simulink model "mdaqdemos_rc_controller"  (R2013a)
settings: Solver=FixedStepDiscrete  SolverMode=SingleTasking  StartTime=0.0  StopTime=inf  FixedStep=0.001  RelTol=1e-3
libraries: microdaq_lib x2
settings Model: SimulationMode=external  Creator=skibool  LastModifiedBy=skibool
settings OptimizationCC: OptimizeModelRefInitCode=on  LifeSpan=1
settings DebuggingCC: UnderspecifiedInitializationDetection=Simplified  StateNameClashWarn=none
settings HardwareCC: ProdBitPerLong=40  ProdLargestAtomicInteger=Integer  ProdIntDivRoundTo=Zero  ProdEndianess=LittleEndian  ProdHWDeviceType=Texas Instruments->C6000
settings RTWCC: SystemTargetFile=microdaq.tlc  TemplateMakefile=microdaq.tmf  PostCodeGenCommand=microdaq_postcodegen(buildInfo)  Description=MicroDAQ Real-Time Measurement System  ProcessScript=microdaq_make_rtw_hook
settings CodeAppCC: IgnoreCustomStorageClasses=off
settings STFCustomTargetCC: CodeReplacementLibrary=TI C674x  CombineOutputUpdateFcns=on  ERTCustomFileBanners=on  SupportContinuousTime=off  SupportNonInlinedSFcns=off  MATLABClassNameForMDSCustomization=Simulink.SoftwareTarget.ERTCustomization  SystemTargetFile=microdaq.tlc
settings ERTTargetCC: CodeReplacementLibrary=TI C674x  GenerateSampleERTMain=off  ParMdlRefBuildCompliant=off  CompOptLevelCompliant=off  ConcurrentExecutionCompliant=off  ERTFirstTimeCompliant=off  ModelStepFunctionPrototypeControlCompliant=off  CPPClassGenCompliant=off  ExtMode=on  ExtModeStaticAlloc=on  ExtModeStaticAllocSize=10485760  ExtModeMexArgs=getpref('microdaq','TargetIP') 1 4344  ERTCustomFileTemplate=microdaq_main.tlc

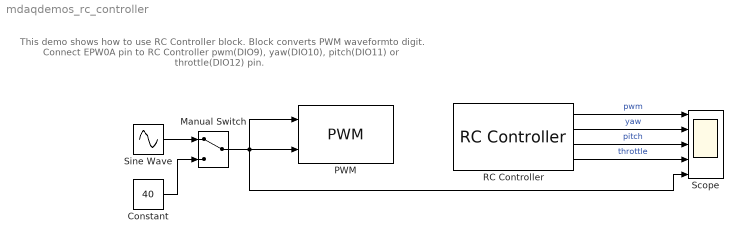
== system mdaqdemos_rc_controller ==
  note: This demo shows how to use RC Controller block. Block converts PWM waveformto digit.
      | Connect EPW0A pin to RC Controller pwm(DIO9), yaw(DIO10), pitch(DIO11) or throttle(DIO12) pin.
  Constant : Constant  Value=40
  Manual Switch : ManualSwitch
  PWM : microdaq_lib/PWM  pModule=EPWM0  pMode=PERIOD  pPeriod=2000  pPolarity=Active HIGH  SampleTime=-1
  RC Controller : microdaq_lib/RC Controller  pPRUnum=PRU0  SampleTime=-1
  Scope : Scope  NumInputPorts=5
      settings: TimeRange=1  YMin=0~0~0~0~0  YMax=1100~1300~1100~1100~50
  Sine Wave : Sin  Amplitude=25  Bias=25  Frequency=20
  wires:
  RC Controller/1 -> Scope/1  "pwm"
  RC Controller/2 -> Scope/2  "yaw"
  RC Controller/3 -> Scope/3  "pitch"
  RC Controller/4 -> Scope/4  "throttle"
  Manual Switch/1 -> Scope/5, PWM/2, PWM/1
  Sine Wave/1 -> Manual Switch/1
  Constant/1 -> Manual Switch/2
